simulink model "power_wind"  (R2014b)
settings: Solver=ode23tb  StartTime=0.0  StopTime=20  MaxStep=1/60  RelTol=1e-4  AbsTol=1e-3
InitFcn:
  | xInitial = init_power_wind_ig;
undefined symbols (not defined in the file): D1, D11, Delta
libraries: powerlib_meascontrol x45, powerlib x29, DRlib x3, factslib x1
(part 1 of 4)
Description:
  | Copyright 2008-2014 The MathWorks, Inc.
settings Model: ExtModeAutoUpdateStatusClock=off  Creator=MathWorks  LastModifiedBy=HPSEDC
settings DataIOCC: LoadInitialState=on  SignalLoggingSaveFormat=ModelDataLogs  SaveOutput=off  SaveTime=off  SignalLoggingName=logsOut
settings OptimizationCC: ExpressionDepthLimit=2147483647  InitFltsAndDblsToZero=on
settings DebuggingCC: UnderspecifiedInitializationDetection=Classic  MergeDetectMultiDrivingBlocksExec=none  CheckExecutionContextPreStartOutputMsg=on  CheckExecutionContextRuntimeOutputMsg=on  SignalResolutionControl=TryResolveAllWithWarning  MultiTaskDSMMsg=warning  MultiTaskCondExecSysMsg=none  FcnCallInpInsideContextMsg=UseLocalSettings  StateNameClashWarn=warning  InitInArrayFormatMsg=none
settings RTWCC: IncludeERTFirstTime=on
settings GRTTargetCC: CombineOutputUpdateFcns=off  GRTInterface=on

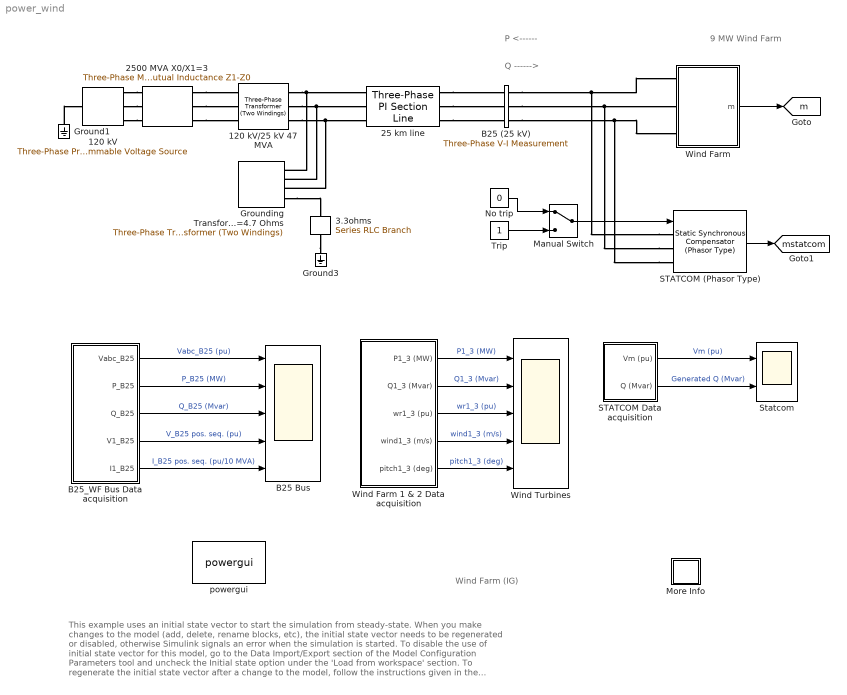
== system power_wind ==
  note: This example uses an initial state vector to start the simulation from steady-state. When you make changes to the model (add, delete, rename blocks, etc),
      | the initial state vector needs to be regenerated or disabled, otherwise Simulink signals an error when the simulation is started.
      | To disable the use of initial state vector for this model, go to the Data Import/Export section of the Model Configuration Parameters tool and uncheck the
      | Initial state option under the 'Load from workspace' section.
      | To regenerate the initial state vector after a change to the model, follow the instructions given in the initialization file for this model.
      | Type open('init_power_wind_ig') at the matlab prompt to view this file.
  note: Wind Farm (IG)
  note: P
      | <------
  note: Q
      | ------>
  note: 9 MW Wind Farm
  " Wind Turbines" : Scope  NumInputPorts=5
  120 kV : powerlib/Electrical Sources/Three-Phase Programmable Voltage Source  PositiveSequence=[120e3 0 60]  VariationEntity=None  VariationType=Table of time-amplitude pairs  VariationTypeAlt=Step  VariationStep=-0.15  VariationRate=10  VariationMagnitude=0.3  VariationFrequency=2  VariationTiming=[5 5.5]  VariationPhaseA=off  Amplitudes="[1.0  0.5  1.0 ]"  TimeValues="[0  10  10.1]"  HarmonicGeneration=off  HarmonicA=[1 -0.1 0 1]  HarmonicB=[2 0.15 35 2]  Timing="[5  5.5]"  BusType=swing  Pref=1e3  Qref=0  Qmin=-inf  Qmax=inf
  120 kV/25 kV 47 MVA : powerlib/Elements/Three-Phase Transformer (Two Windings)  Winding1Connection=Yg  UNITS=pu  NominalPower=[47e6 60 ]  Winding1="[ 120e3  0.08/30   0.08 ]"  Winding2Connection=Delta (D1)  Winding2="[ 25e3  0.08/30  0.08]"  SetSaturation=off  Rm=500  Lm=500  Saturation="[ 0,0  ;  0.005,1.2  ;  1.0,1.4 ]"  Hysteresis=off  DataFile='basic_model'  SetInitialFlux=off  InitialFluxes=[ 0.8 , -0.8 , 0.7 ]  Measurements=None  MoreParameters=off  BreakLoop=off  DataType=off  TransfoNumber=0
  25 km line : powerlib/Elements/Three-Phase PI Section Line  LConnTagsString=a|b|c  RConnTagsString=A|B|C  Frequency=60  Resistances=[0.1153 0.413]  Inductances=[1.05e-3 3.32e-3]  Capacitances=[11.33e-009 5.01e-009]  Length=25
  2500 MVA X0/X1=3 : powerlib/Elements/Three-Phase Mutual Inductance Z1-Z0  LConnTagsString=a|b|c  RConnTagsString=A|B|C  PositiveSequence="[0.1  1.0/(2*pi*60)] *120e3^2/2500e6"  ZeroSequence="[0.3  3.0/(2*pi*60)] *120e3^2/2500e6"
  "3.3ohms " : powerlib/Elements/Series RLC Branch  LConnTagsString=__new0  RConnTagsString=__new0  BranchType=R  Resistance=3.3  Inductance=1.0  SetiL0=off  InitialCurrent=0  Capacitance=1.0  Setx0=off  InitialVoltage=0  Measurements=None
  B25 (25 kV) : powerlib/Measurements/Three-Phase V-I Measurement  VoltageMeasurement=phase-to-ground  SetLabelV=on  LabelV=Vabc_B25  Vpu=on  VpuLL=off  CurrentMeasurement=yes  SetLabelI=on  LabelI=Iabc_B25  Ipu=on  Pbase=10e6  Vbase=25e3  OutputType=Complex  PhasorSimulation=on  PSBequivalent=0
  B25 Bus : Scope  NumInputPorts=5
  B25_WF Bus Data acquisition : Subsystem
  Ground1 : powerlib/Elements/Ground  LConnTagsString=a
  Ground3 : powerlib/Elements/Ground  LConnTagsString=a
  Grounding Transformer X0=4.7 Ohms : powerlib/Elements/Three-Phase Transformer (Two Windings)  Winding1Connection=Yn  UNITS=pu  NominalPower=[100e6 60]  Winding1="[ 25e3  4.7/(25e3^2/100e6)/30    4.7/(25e3^2/100e6)]"  Winding2Connection=Delta (D11)  Winding2="[ 25e3  1e-6  0]"  SetSaturation=off  Rm=500  Lm=500  Saturation="[ 0,0  ;  0.005,1.2  ;  1.0,1.4 ]"  Hysteresis=off  DataFile='basic_model'  SetInitialFlux=off  InitialFluxes=[ 0.8 , -0.8 , 0.7 ]  Measurements=None  MoreParameters=off  BreakLoop=off  DataType=off  TransfoNumber=0
  Manual Switch : ManualSwitch
  More Info : Subsystem
      settings: OpenFcn=showdemo(bdroot(gcb))
      mask Display: disp('?')
  No trip : Constant  Value=0
  STATCOM (Phasor Type) : factslib/Power-Electronics Based FACTS/Static Synchronous Compensator (Phasor Type)  ShowParameters=Power data  SystemNominal=[ 25e3, 60 ]  Pnom_SH=3e6  RL_SH=[ 0.22/30, 0.22 ]  Iinit_SH=[0, 0 ]  VnomDC=40000/10  C_DC=375e-6*(3/100)*10^2  OpMode_SH=Voltage regulation  ExternalVref=off  Vref_SH=1.00  MaxRateChangeVref_SH=10  Droop_SH=0.03  Par_VacReg=[5 1000]  Qref_SH=0  MaxRateChangeQref_SH=2  Par_VdcReg=[0.1e-3 20e-3]  Par_IReg_SH=[0.3 10 0.22]
  STATCOM Data acquisition : Subsystem
  Statcom : Scope  NumInputPorts=2
  Trip : Constant
  Wind Farm : Subsystem
      mask Display:
      | plot(0,0,118,100)
      | plot([56 62],[4 4],[56 57],[4 52],[62 61],[4 52])
      | plot([57 59 61],[52 52.5 52])
      | plot([61 61.5 62 63 63],[52 52.2 52.5 54 56])
      | plot([63 59 57.6 57.3 56 55],[56 58 57.8 55.6 54.2 54])
      | plot([55 57],[54 52],[57.3 63],[55.6 54])
      | plot([57.6 57 55 54.7 60 81],[57.6 57.3 58 59.4 64 82])
      | plot([81 83 84 84.2 83 81],[82 83.6 83.4 83 80.8 78.7])
      | plot([81 60.5 57.6],[78.7 60 57.6])
      | plot([54.7 53 51 51.3 52.5],[59.4 58.8 58 56 55])
      | plot([52.5 53.7 54.5 55],[55 54.9 54.6 54])
      | plot([51 47 35 33 32 33 35],[58 59 66 67.7 68.5 68.4 68])
      | plot([35 45 52 53 53.7],[68 64 61 60 59.2])
      | plot([52.5 51 50.8 51.5 55],[55 26 21 26 54])
  Wind Farm 1 & 2 Data acquisition : Subsystem
  powergui : powerlib/powergui  Priority=2  SimulationMode=Phasor  SolverType=Tustin  SampleTime=0  frequency=60  SPID=off  DisableSnubberDevices=off  DisableRonSwitches=off  DisableVfSwitches=off  SwTol=0  DisplayEquations=off  Interpol=off  methode=off  Ts=0  frequencyindice=60  Pbase=100e6  ErrMax=1e-4  Iterations=50  UnitsV=kV  UnitsW=MW  FunctionMessages=off  echomessages=off  HookPort=off  EnableUseOfTLC=off  x0status=blocks  RestoreLinks=no  ResistiveCurrentMeasurement=off  Frange=[0:2:500]  Ylog=off  Xlog=off  ShowGrid=off  save=off  variable=ZData  structure=0  ZoomFFT=on  StartTime=0.0  cycles=1  DisplayStyle=1  fundamental=60  FreqAxis=off  MaxFrequency=1000  frequencyindicesteady=1  RmsSteady=1  display=off
  tag scope: m=global, mstatcom=global
  wires:
  B25_WF Bus Data acquisition/1("Vabc_B25 ") -> B25 Bus/1  "Vabc_B25 (pu)"
  B25_WF Bus Data acquisition/2(P_B25) -> B25 Bus/2  "P_B25 (MW)"
  B25_WF Bus Data acquisition/3(Q_B25) -> B25 Bus/3  "Q_B25 (Mvar)"
  B25_WF Bus Data acquisition/4(V1_B25) -> B25 Bus/4  "V_B25 pos. seq. (pu)"
  B25_WF Bus Data acquisition/5(I1_B25) -> B25 Bus/5  "I_B25 pos. seq. (pu/10 MVA)"
  Wind Farm/1(m) -> [m]
  No trip/1 -> Manual Switch/1
  Trip/1 -> Manual Switch/2
  STATCOM Data acquisition/1(Vm (pu)) -> Statcom/1  "Vm (pu)"
  STATCOM Data acquisition/2(Q (Mvar)) -> Statcom/2  "Generated Q (Mvar)"
  Wind Farm 1 & 2 Data acquisition/1(P1_3 (MW)) -> " Wind Turbines"/1  "P1_3 (MW)"
  Wind Farm 1 & 2 Data acquisition/2(Q1_3 (Mvar)) -> " Wind Turbines"/2  "Q1_3 (Mvar)"
  Wind Farm 1 & 2 Data acquisition/3(wr1_3 (pu)) -> " Wind Turbines"/3  "wr1_3 (pu)"
  Wind Farm 1 & 2 Data acquisition/4(wind1_3 (m/s)) -> " Wind Turbines"/4  "wind1_3 (m/s)"
  Wind Farm 1 & 2 Data acquisition/5(pitch1_3 (deg)) -> " Wind Turbines"/5  "pitch1_3 (deg)"
  Manual Switch/1 -> STATCOM (Phasor Type)/1
  STATCOM (Phasor Type)/1 -> [mstatcom]
  connections:
  120 kV/25 kV 47 MVA/RConn2 -- 25 km line/LConn2 -- Grounding Transformer X0=4.7 Ohms/LConn2
  120 kV/25 kV 47 MVA/RConn3 -- 25 km line/LConn3 -- Grounding Transformer X0=4.7 Ohms/LConn3
  120 kV/25 kV 47 MVA/RConn1 -- 25 km line/LConn1 -- Grounding Transformer X0=4.7 Ohms/LConn1
  STATCOM (Phasor Type)/LConn2 -- B25 (25 kV)/RConn2 -- Wind Farm/LConn2
  STATCOM (Phasor Type)/LConn3 -- B25 (25 kV)/RConn3 -- Wind Farm/LConn3
  Ground1/LConn1 -- 120 kV/LConn1
  120 kV/RConn1 -- 2500 MVA X0/X1=3/LConn1
  120 kV/RConn2 -- 2500 MVA X0/X1=3/LConn2
  120 kV/RConn3 -- 2500 MVA X0/X1=3/LConn3
  "3.3ohms "/RConn1 -- Ground3/LConn1
  Grounding Transformer X0=4.7 Ohms/LConn4 -- "3.3ohms "/LConn1
  2500 MVA X0/X1=3/RConn1 -- 120 kV/25 kV 47 MVA/LConn1
  2500 MVA X0/X1=3/RConn2 -- 120 kV/25 kV 47 MVA/LConn2
  2500 MVA X0/X1=3/RConn3 -- 120 kV/25 kV 47 MVA/LConn3
  STATCOM (Phasor Type)/LConn1 -- B25 (25 kV)/RConn1 -- Wind Farm/LConn1
  25 km line/RConn1 -- B25 (25 kV)/LConn1
  25 km line/RConn2 -- B25 (25 kV)/LConn2
  25 km line/RConn3 -- B25 (25 kV)/LConn3

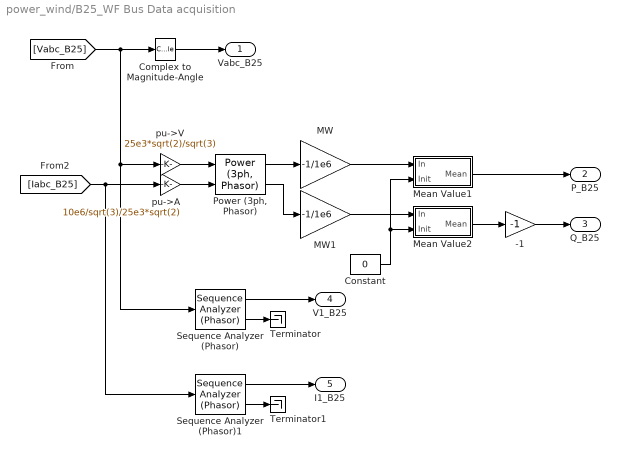
== system power_wind/B25_WF Bus Data acquisition ==
  -1 : Gain  Gain=-1  SaturateOnIntegerOverflow=on  OutDataTypeStr=Inherit: Same as input  ParamDataTypeStr=Inherit: Same as input
  "Complex to Magnitude-Angle " : ComplexToMagnitudeAngle  Output=Magnitude
  Constant : Constant  Value=0
  MW : Gain  Gain=-1/1e6  SaturateOnIntegerOverflow=on  OutDataTypeStr=Inherit: Same as input  ParamDataTypeStr=Inherit: Same as input
  MW1 : Gain  Gain=-1/1e6  SaturateOnIntegerOverflow=on  OutDataTypeStr=Inherit: Same as input  ParamDataTypeStr=Inherit: Same as input
  Mean Value1 : Subsystem  mask(Mean value){Period=1/60}
      mask prompts: Period "Averaging period (s):"
      mask help: This block uses the running window averaging technique to compute the mean value of the input signal over the specified period.
  Mean Value2 : Subsystem  mask(Mean value){Period=1/60}
      mask prompts: Period "Averaging period (s):"
      mask help: This block uses the running window averaging technique to compute the mean value of the input signal over the specified period.
  "Power (3ph, Phasor)" : powerlib_meascontrol/Measurements/Power (3ph, Phasor)
  Sequence Analyzer (Phasor) : powerlib_meascontrol/Measurements/Sequence Analyzer (Phasor)  seq=Positive
  Sequence Analyzer (Phasor)1 : powerlib_meascontrol/Measurements/Sequence Analyzer (Phasor)  seq=Positive
  Terminator : Terminator
  Terminator1 : Terminator
  pu->A : Gain  Gain=10e6/sqrt(3)/25e3*sqrt(2)  SaturateOnIntegerOverflow=on  OutDataTypeStr=Inherit: Same as input  ParamDataTypeStr=Inherit: Same as input
  pu->V : Gain  Gain=25e3*sqrt(2)/sqrt(3)  SaturateOnIntegerOverflow=on  OutDataTypeStr=Inherit: Same as input  ParamDataTypeStr=Inherit: Same as input
  "Vabc_B25 " : Outport
  P_B25 : Outport  Port=2
  Q_B25 : Outport  Port=3
  V1_B25 : Outport  Port=4
  I1_B25 : Outport  Port=5
  wires:
  pu->A/1 -> "Power (3ph, Phasor)"/2
  pu->V/1 -> "Power (3ph, Phasor)"/1
  "Power (3ph, Phasor)"/1 -> MW/1
  "Complex to Magnitude-Angle "/1 -> "Vabc_B25 "/1
  [Vabc_B25] -> Sequence Analyzer (Phasor)/1, pu->V/1, "Complex to Magnitude-Angle "/1
  [Iabc_B25] -> Sequence Analyzer (Phasor)1/1, pu->A/1
  MW/1 -> Mean Value1/1(In)
  MW1/1 -> Mean Value2/1(In)
  Constant/1 -> Mean Value1/2(Init), Mean Value2/2(Init)
  Mean Value1/1(Mean) -> P_B25/1
  Mean Value2/1(Mean) -> -1/1
  Sequence Analyzer (Phasor)/1 -> V1_B25/1
  Sequence Analyzer (Phasor)/2 -> Terminator/1
  Sequence Analyzer (Phasor)1/1 -> I1_B25/1
  Sequence Analyzer (Phasor)1/2 -> Terminator1/1
  -1/1 -> Q_B25/1
  "Power (3ph, Phasor)"/2 -> MW1/1

== system power_wind/More Info ==

== system power_wind/STATCOM Data acquisition ==
  Bus Selector : BusSelector  OutputSignals=Control.Vm (pu),Control.Qm (pu)
  pu->Mvar : Gain  Gain=-3e6/1e6  SaturateOnIntegerOverflow=on  OutDataTypeStr=Inherit: Same as input  ParamDataTypeStr=Inherit: Same as input
  Vm (pu) : Outport
  Q (Mvar) : Outport  Port=2
  wires:
  Bus Selector/1 -> Vm (pu)/1  "<Vm (pu)>"
  Bus Selector/2 -> pu->Mvar/1  "<Qm (pu)>"
  pu->Mvar/1 -> Q (Mvar)/1  "Generated Q (Mvar)"
  [mstatcom] -> Bus Selector/1

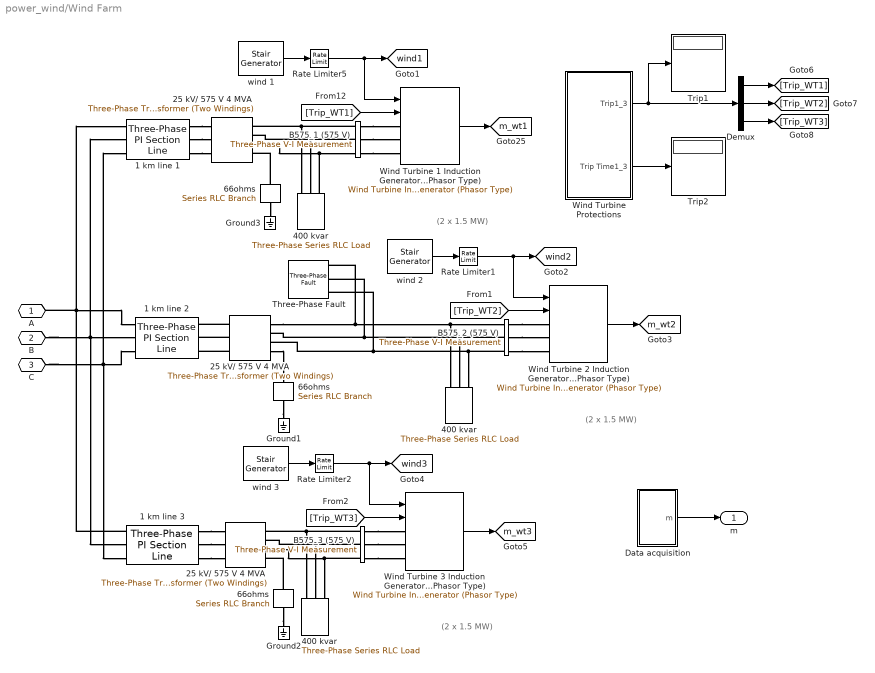
== system power_wind/Wind Farm ==
  note: (2 x 1.5 MW)
  note: (2 x 1.5 MW)
  note: (2 x 1.5 MW)
  " 66ohms " : powerlib/Elements/Series RLC Branch  LConnTagsString=__new0  RConnTagsString=__new0  BranchType=R  Resistance=66  Inductance=1.0  SetiL0=off  InitialCurrent=0  Capacitance=1.0  Setx0=off  InitialVoltage=0  Measurements=None
  "1 km line 1 " : powerlib/Elements/Three-Phase PI Section Line  LConnTagsString=a|b|c  RConnTagsString=A|B|C  Frequency=60  Resistances=[0.1153 0.413]  Inductances=[1.05e-3 3.32e-3]  Capacitances=[11.33e-009 5.01e-009]  Length=1
  1 km line 2 : powerlib/Elements/Three-Phase PI Section Line  LConnTagsString=a|b|c  RConnTagsString=A|B|C  Frequency=60  Resistances=[0.1153 0.413]  Inductances=[1.05e-3 3.32e-3]  Capacitances=[11.33e-009 5.01e-009]  Length=1
  1 km line 3 : powerlib/Elements/Three-Phase PI Section Line  LConnTagsString=a|b|c  RConnTagsString=A|B|C  Frequency=60  Resistances=[0.1153 0.413]  Inductances=[1.05e-3 3.32e-3]  Capacitances=[11.33e-009 5.01e-009]  Length=1
  25 kV/ 575 V 4 MVA : powerlib/Elements/Three-Phase Transformer (Two Windings)  Winding1Connection=Yg  UNITS=pu  NominalPower="[4e6  60]"  Winding1=[25e3 , 0.025/30 , 0.025]  Winding2Connection=Yn  Winding2=[ 575, 0.025/30 , 0.025]  SetSaturation=off  Rm=500  Lm=inf  Saturation=[ 0,0 ; 0.0024,1.2 ; 1.0,1.52 ]  Hysteresis=off  DataFile='hysteresis'  SetInitialFlux=off  InitialFluxes=[ 0.8 , -0.8 , 0.7 ]  Measurements=None  MoreParameters=off  BreakLoop=off  DataType=off  TransfoNumber=0
  "25 kV/ 575 V 4 MVA " : powerlib/Elements/Three-Phase Transformer (Two Windings)  Winding1Connection=Yg  UNITS=pu  NominalPower="[4e6  60]"  Winding1=[25e3 , 0.025/30 , 0.025]  Winding2Connection=Yn  Winding2=[ 575, 0.025/30 , 0.025]  SetSaturation=off  Rm=500  Lm=inf  Saturation=[ 0,0 ; 0.0024,1.2 ; 1.0,1.52 ]  Hysteresis=off  DataFile='hysteresis'  SetInitialFlux=off  InitialFluxes=[ 0.8 , -0.8 , 0.7 ]  Measurements=None  MoreParameters=off  BreakLoop=off  DataType=off  TransfoNumber=0
  "25 kV/ 575 V 4 MVA  " : powerlib/Elements/Three-Phase Transformer (Two Windings)  Winding1Connection=Yg  UNITS=pu  NominalPower="[4e6  60]"  Winding1=[25e3 , 0.025/30 , 0.025]  Winding2Connection=Yn  Winding2=[ 575, 0.025/30 , 0.025]  SetSaturation=off  Rm=500  Lm=inf  Saturation=[ 0,0 ; 0.0024,1.2 ; 1.0,1.52 ]  Hysteresis=off  DataFile='hysteresis'  SetInitialFlux=off  InitialFluxes=[ 0.8 , -0.8 , 0.7 ]  Measurements=None  MoreParameters=off  BreakLoop=off  DataType=off  TransfoNumber=0
  400 kvar : powerlib/Elements/Three-Phase Series RLC Load  LConnTagsString=A|B|C  Configuration=Delta  NominalVoltage=575  NominalFrequency=60  ActivePower=0  InductivePower=0  CapacitivePower=400e3  Measurements=None  LoadType=constant Z
  "400 kvar " : powerlib/Elements/Three-Phase Series RLC Load  LConnTagsString=A|B|C  Configuration=Delta  NominalVoltage=575  NominalFrequency=60  ActivePower=0  InductivePower=0  CapacitivePower=400e3  Measurements=None  LoadType=constant Z
  "400 kvar  " : powerlib/Elements/Three-Phase Series RLC Load  LConnTagsString=A|B|C  Configuration=Delta  NominalVoltage=575  NominalFrequency=60  ActivePower=0  InductivePower=0  CapacitivePower=400e3  Measurements=None  LoadType=constant Z
  "66ohms " : powerlib/Elements/Series RLC Branch  LConnTagsString=__new0  RConnTagsString=__new0  BranchType=R  Resistance=66  Inductance=1.0  SetiL0=off  InitialCurrent=0  Capacitance=1.0  Setx0=off  InitialVoltage=0  Measurements=None
  "66ohms  " : powerlib/Elements/Series RLC Branch  LConnTagsString=__new0  RConnTagsString=__new0  BranchType=R  Resistance=66  Inductance=1.0  SetiL0=off  InitialCurrent=0  Capacitance=1.0  Setx0=off  InitialVoltage=0  Measurements=None
  B575_1 (575 V) : powerlib/Measurements/Three-Phase V-I Measurement  VoltageMeasurement=phase-to-ground  SetLabelV=on  LabelV=Vabc_B575_1  Vpu=on  VpuLL=off  CurrentMeasurement=yes  SetLabelI=on  LabelI=Iabc_B575_1  Ipu=on  Pbase=2*1.5e6/0.9  Vbase=575  OutputType=Complex  PhasorSimulation=on  PSBequivalent=0
  B575_2 (575 V) : powerlib/Measurements/Three-Phase V-I Measurement  VoltageMeasurement=phase-to-ground  SetLabelV=on  LabelV=Vabc_B575_2  Vpu=on  VpuLL=off  CurrentMeasurement=yes  SetLabelI=on  LabelI=Iabc_B575_2  Ipu=on  Pbase=2*1.5e6/0.9  Vbase=575  OutputType=Complex  PhasorSimulation=on  PSBequivalent=0
  B575_3 (575 V) : powerlib/Measurements/Three-Phase V-I Measurement  VoltageMeasurement=phase-to-ground  SetLabelV=on  LabelV=Vabc_B575_3  Vpu=on  VpuLL=off  CurrentMeasurement=yes  SetLabelI=on  LabelI=Iabc_B575_3  Ipu=on  Pbase=2*1.5e6/0.9  Vbase=575  OutputType=Complex  PhasorSimulation=on  PSBequivalent=0
  Data acquisition : Subsystem
  Demux : Demux  Outputs=3
  Ground1 : powerlib/Elements/Ground  LConnTagsString=a
  Ground2 : powerlib/Elements/Ground  LConnTagsString=a
  Ground3 : powerlib/Elements/Ground  LConnTagsString=a
  Rate Limiter1 : RateLimiter
  Rate Limiter2 : RateLimiter
  Rate Limiter5 : RateLimiter
  Three-Phase Fault : powerlib/Elements/Three-Phase Fault  InitialStates=0  FaultA=on  FaultB=on  FaultC=off  GroundFault=on  SwitchTimes=[ 15 15.1]  External=off  SwitchStatus=NaN  FaultResistance=0.001  GroundResistance=0.001  SnubberResistance=1e6  SnubberCapacitance=inf  Measurements=None
  Trip1 : Display
  Trip2 : Display
  Wind Turbine Protections : Subsystem
  Wind Turbine 1 Induction Generator (Phasor Type) : DRlib/Wind Generation/Wind Turbine Induction Generator (Phasor Type)  ShowParameters=Turbine data  nom=[2*1.5e6/0.9 575 60]  sta=[ 0.004843 0.1248]  rot=[ 0.004377 0.1791]  Lm=6.77  mec=[5.04 0.01 3]  init="[ -0.01,0   0,0,0   0,0,0 ]"  ExternalTm=off  DisplayTurbChar=off  pitch_angle=0  Pmec=2*1.5e6  wind_base=9  P_wind_base=1  speed_nom=1  K_pitch_gain=[5 25]  pitch_max=45  pitch_rate=2
  Wind Turbine 2 Induction Generator (Phasor Type) : DRlib/Wind Generation/Wind Turbine Induction Generator (Phasor Type)  ShowParameters=Turbine data  nom=[2*1.5e6/0.9 575 60]  sta=[ 0.004843 0.1248]  rot=[ 0.004377 0.1791]  Lm=6.77  mec=[5.04 0.01 3]  init="[ -0.01,0   0,0,0   0,0,0 ]"  ExternalTm=off  DisplayTurbChar=off  pitch_angle=0  Pmec=2*1.5e6  wind_base=9  P_wind_base=1  speed_nom=1  K_pitch_gain=[5 25]  pitch_max=45  pitch_rate=2
  Wind Turbine 3 Induction Generator (Phasor Type) : DRlib/Wind Generation/Wind Turbine Induction Generator (Phasor Type)  ShowParameters=Turbine data  nom=[2*1.5e6/0.9 575 60]  sta=[ 0.004843 0.1248]  rot=[ 0.004377 0.1791]  Lm=6.77  mec=[5.04 0.01 3]  init="[ -0.01,0   0,0,0   0,0,0 ]"  ExternalTm=off  DisplayTurbChar=off  pitch_angle=0  Pmec=2*1.5e6  wind_base=9  P_wind_base=1  speed_nom=1  K_pitch_gain=[5 25]  pitch_max=45  pitch_rate=2
  wind 1 : powerlib_meascontrol/Pulse & Signal Generators/Stair Generator  t=[ 0 2]  e=[8 11]  Ts=0
  wind 2 : powerlib_meascontrol/Pulse & Signal Generators/Stair Generator  t=[ 0 4]  e=[8 11]  Ts=0
  wind 3 : powerlib_meascontrol/Pulse & Signal Generators/Stair Generator  t=[ 0 6]  e=[8 11]  Ts=0
  A : PMIOPort  Port=1  Side=Left
  B : PMIOPort  Port=2  Side=Left
  C : PMIOPort  Port=3  Side=Left
  m : Outport
  tag scope: m_wt1=global, m_wt2=global, m_wt3=global, wind1=global, wind2=global, wind3=global
  wires:
  Data acquisition/1(m) -> m/1
  Wind Turbine 1 Induction Generator (Phasor Type)/1 -> [m_wt1]
  Rate Limiter5/1 -> [wind1], Wind Turbine 1 Induction Generator (Phasor Type)/1
  wind 1/1 -> Rate Limiter5/1
  [Trip_WT1] -> Wind Turbine 1 Induction Generator (Phasor Type)/2
  Wind Turbine 2 Induction Generator (Phasor Type)/1 -> [m_wt2]
  Rate Limiter1/1 -> Wind Turbine 2 Induction Generator (Phasor Type)/1, [wind2]
  wind 2/1 -> Rate Limiter1/1
  [Trip_WT2] -> Wind Turbine 2 Induction Generator (Phasor Type)/2
  Wind Turbine 3 Induction Generator (Phasor Type)/1 -> [m_wt3]
  Rate Limiter2/1 -> [wind3], Wind Turbine 3 Induction Generator (Phasor Type)/1
  wind 3/1 -> Rate Limiter2/1
  [Trip_WT3] -> Wind Turbine 3 Induction Generator (Phasor Type)/2
  Wind Turbine Protections/1(Trip1_3) -> Trip1/1, Demux/1
  Demux/1 -> [Trip_WT1]
  Wind Turbine Protections/2(Trip Time1_3) -> Trip2/1
  Demux/2 -> [Trip_WT2]
  Demux/3 -> [Trip_WT3]
  connections:
  B575_1 (575 V)/RConn3 -- Wind Turbine 1 Induction Generator (Phasor Type)/LConn3
  B575_1 (575 V)/RConn2 -- Wind Turbine 1 Induction Generator (Phasor Type)/LConn2
  B575_1 (575 V)/RConn1 -- Wind Turbine 1 Induction Generator (Phasor Type)/LConn1
  400 kvar/LConn3 -- B575_1 (575 V)/LConn3 -- 25 kV/ 575 V 4 MVA/RConn3
  25 kV/ 575 V 4 MVA/RConn2 -- 400 kvar/LConn2 -- B575_1 (575 V)/LConn2
  25 kV/ 575 V 4 MVA/RConn1 -- 400 kvar/LConn1 -- B575_1 (575 V)/LConn1
  "1 km line 1 "/RConn3 -- 25 kV/ 575 V 4 MVA/LConn3
  "1 km line 1 "/RConn2 -- 25 kV/ 575 V 4 MVA/LConn2
  "1 km line 1 "/RConn1 -- 25 kV/ 575 V 4 MVA/LConn1
  Three-Phase Fault/LConn3 -- "400 kvar "/LConn3 -- B575_2 (575 V)/LConn3 -- "25 kV/ 575 V 4 MVA "/RConn3
  Three-Phase Fault/LConn2 -- "400 kvar "/LConn2 -- B575_2 (575 V)/LConn2 -- "25 kV/ 575 V 4 MVA "/RConn2
  Three-Phase Fault/LConn1 -- "25 kV/ 575 V 4 MVA "/RConn1 -- "400 kvar "/LConn1 -- B575_2 (575 V)/LConn1
  B575_2 (575 V)/RConn3 -- Wind Turbine 2 Induction Generator (Phasor Type)/LConn3
  B575_2 (575 V)/RConn2 -- Wind Turbine 2 Induction Generator (Phasor Type)/LConn2
  B575_2 (575 V)/RConn1 -- Wind Turbine 2 Induction Generator (Phasor Type)/LConn1
  "25 kV/ 575 V 4 MVA "/LConn3 -- 1 km line 2/RConn3
  "25 kV/ 575 V 4 MVA "/LConn2 -- 1 km line 2/RConn2
  "25 kV/ 575 V 4 MVA "/LConn1 -- 1 km line 2/RConn1
  B575_3 (575 V)/LConn3 -- "400 kvar  "/LConn3 -- "25 kV/ 575 V 4 MVA  "/RConn3
  "25 kV/ 575 V 4 MVA  "/RConn2 -- "400 kvar  "/LConn2 -- B575_3 (575 V)/LConn2
  "25 kV/ 575 V 4 MVA  "/RConn1 -- "400 kvar  "/LConn1 -- B575_3 (575 V)/LConn1
  B575_3 (575 V)/RConn3 -- Wind Turbine 3 Induction Generator (Phasor Type)/LConn3
  B575_3 (575 V)/RConn2 -- Wind Turbine 3 Induction Generator (Phasor Type)/LConn2
  B575_3 (575 V)/RConn1 -- Wind Turbine 3 Induction Generator (Phasor Type)/LConn1
  1 km line 3/RConn3 -- "25 kV/ 575 V 4 MVA  "/LConn3
  1 km line 3/RConn2 -- "25 kV/ 575 V 4 MVA  "/LConn2
  1 km line 3/RConn1 -- "25 kV/ 575 V 4 MVA  "/LConn1
  1 km line 3/LConn1 -- A/RConn1 -- "1 km line 1 "/LConn1 -- 1 km line 2/LConn1
  B/RConn1 -- "1 km line 1 "/LConn2 -- 1 km line 3/LConn2 -- 1 km line 2/LConn2
  C/RConn1 -- "1 km line 1 "/LConn3 -- 1 km line 3/LConn3 -- 1 km line 2/LConn3
  "66ohms "/RConn1 -- Ground3/LConn1
  "66ohms  "/RConn1 -- Ground1/LConn1
  "25 kV/ 575 V 4 MVA "/RConn4 -- "66ohms  "/LConn1
  " 66ohms "/RConn1 -- Ground2/LConn1
  " 66ohms "/LConn1 -- "25 kV/ 575 V 4 MVA  "/RConn4
  "66ohms "/LConn1 -- 25 kV/ 575 V 4 MVA/RConn4

== system power_wind/Wind Farm 1 & 2 Data acquisition ==
  -1 : Gain  Gain=-1  SaturateOnIntegerOverflow=on  OutDataTypeStr=Inherit: Same as input  ParamDataTypeStr=Inherit: Same as input
  Bus Selector1 : BusSelector  OutputSignals=P1_3 (MW),Q1_3 (Mvar),wr1_3,wind1_3 (m_s),pitch1_3
  Constant1 : Constant  Value=0
  Mean Value3 : Subsystem  mask(Mean value){Period=1/60}
      mask prompts: Period "Averaging period (s):"
      mask help: This block uses the running window averaging technique to compute the mean value of the input signal over the specified period.
  Mean Value4 : Subsystem  mask(Mean value){Period=1/60}
      mask prompts: Period "Averaging period (s):"
      mask help: This block uses the running window averaging technique to compute the mean value of the input signal over the specified period.
  P1_3 (MW) : Outport
  Q1_3 (Mvar) : Outport  Port=2
  wr1_3 (pu) : Outport  Port=3
  wind1_3 (m/s) : Outport  Port=4
  pitch1_3 (deg) : Outport  Port=5
  wires:
  [m] -> Bus Selector1/1
  Constant1/1 -> Mean Value4/2(Init), Mean Value3/2(Init)
  Mean Value4/1(Mean) -> -1/1
  Mean Value3/1(Mean) -> P1_3 (MW)/1
  -1/1 -> Q1_3 (Mvar)/1
  Bus Selector1/1 -> Mean Value3/1(In)  "<P1_3 (MW)>"
  Bus Selector1/2 -> Mean Value4/1(In)  "<Q1_3 (Mvar)>"
  Bus Selector1/3 -> wr1_3 (pu)/1  "<wr1_3>"
  Bus Selector1/4 -> wind1_3 (m/s)/1  "<wind1_3 (m_s)>"
  Bus Selector1/5 -> pitch1_3 (deg)/1  "<pitch1_3>"

== system power_wind/B25_WF Bus Data acquisition/Mean Value1 ==
  note: Mean value
  In : Inport
  Init : Inport  Port=2
  Gain : Gain  Gain=1/Period  SaturateOnIntegerOverflow=on  OutDataTypeStr=Inherit: Same as input  ParamDataTypeStr=Inherit: Same as input
  Step : Step  Time=Period+eps  SampleTime=0
  Sum : Sum  Inputs=+-  SaturateOnIntegerOverflow=on  InputSameDT=on  OutDataTypeStr=Inherit: Same as first input
  Switch : Switch  Threshold=0.5  SaturateOnIntegerOverflow=on
  Transport Delay : TransportDelay  DelayTime=Period
  integrator : Integrator
  Mean : Outport
  wires:
  Transport Delay/1 -> Sum/2
  integrator/1 -> Transport Delay/1, Sum/1
  In/1 -> integrator/1
  Sum/1 -> Gain/1
  Gain/1 -> Switch/1
  Switch/1 -> Mean/1
  Step/1 -> Switch/2
  Init/1 -> Switch/3

== system power_wind/B25_WF Bus Data acquisition/Mean Value2 ==
  note: Mean value
  In : Inport
  Init : Inport  Port=2
  Gain : Gain  Gain=1/Period  SaturateOnIntegerOverflow=on  OutDataTypeStr=Inherit: Same as input  ParamDataTypeStr=Inherit: Same as input
  Step : Step  Time=Period+eps  SampleTime=0
  Sum : Sum  Inputs=+-  SaturateOnIntegerOverflow=on  InputSameDT=on  OutDataTypeStr=Inherit: Same as first input
  Switch : Switch  Threshold=0.5  SaturateOnIntegerOverflow=on
  Transport Delay : TransportDelay  DelayTime=Period
  integrator : Integrator
  Mean : Outport
  wires:
  Init/1 -> Switch/3
  Step/1 -> Switch/2
  Switch/1 -> Mean/1
  Gain/1 -> Switch/1
  Sum/1 -> Gain/1
  In/1 -> integrator/1
  integrator/1 -> Sum/1, Transport Delay/1
  Transport Delay/1 -> Sum/2

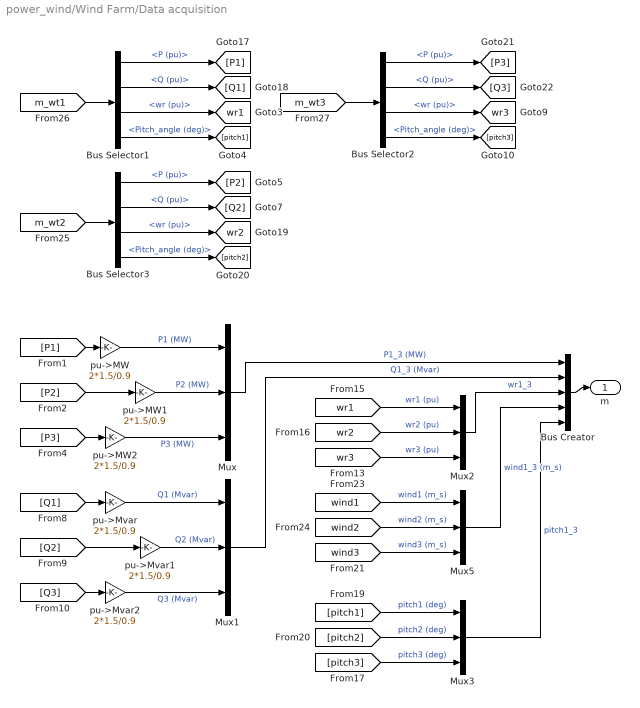
== system power_wind/Wind Farm/Data acquisition ==
  Bus Creator : BusCreator  Inputs=5
  Bus Selector1 : BusSelector  OutputSignals=P (pu),Q (pu),wr (pu),Pitch_angle (deg)
  Bus Selector2 : BusSelector  OutputSignals=P (pu),Q (pu),wr (pu),Pitch_angle (deg)
  Bus Selector3 : BusSelector  OutputSignals=P (pu),Q (pu),wr (pu),Pitch_angle (deg)
  Mux{,1..3,5} (5 alike) : Mux  Inputs=3
  pu->MW : Gain  Gain=2*1.5/0.9  SaturateOnIntegerOverflow=on  OutDataTypeStr=Inherit: Same as input  ParamDataTypeStr=Inherit: Same as input
  pu->MW1 : Gain  Gain=2*1.5/0.9  SaturateOnIntegerOverflow=on  OutDataTypeStr=Inherit: Same as input  ParamDataTypeStr=Inherit: Same as input
  pu->MW2 : Gain  Gain=2*1.5/0.9  SaturateOnIntegerOverflow=on  OutDataTypeStr=Inherit: Same as input  ParamDataTypeStr=Inherit: Same as input
  pu->Mvar : Gain  Gain=2*1.5/0.9  SaturateOnIntegerOverflow=on  OutDataTypeStr=Inherit: Same as input  ParamDataTypeStr=Inherit: Same as input
  pu->Mvar1 : Gain  Gain=2*1.5/0.9  SaturateOnIntegerOverflow=on  OutDataTypeStr=Inherit: Same as input  ParamDataTypeStr=Inherit: Same as input
  pu->Mvar2 : Gain  Gain=2*1.5/0.9  SaturateOnIntegerOverflow=on  OutDataTypeStr=Inherit: Same as input  ParamDataTypeStr=Inherit: Same as input
  m : Outport
  tag scope: wr1=global, wr2=global, wr3=global
  wires:
  [m_wt3] -> Bus Selector2/1
  [m_wt1] -> Bus Selector1/1
  [m_wt2] -> Bus Selector3/1
  Bus Selector1/2 -> [Q1]  "<Q (pu)>"
  Bus Selector1/1 -> [P1]  "<P (pu)>"
  Bus Selector1/4 -> [pitch1]  "<Pitch_angle (deg)>"
  Bus Selector1/3 -> [wr1]  "<wr (pu)>"
  Bus Selector3/4 -> [pitch2]  "<Pitch_angle (deg)>"
  Bus Selector3/3 -> [wr2]  "<wr (pu)>"
  Bus Selector3/2 -> [Q2]  "<Q (pu)>"
  Bus Selector2/4 -> [pitch3]  "<Pitch_angle (deg)>"
  Bus Selector2/3 -> [wr3]  "<wr (pu)>"
  Bus Selector2/2 -> [Q3]  "<Q (pu)>"
  Bus Selector2/1 -> [P3]  "<P (pu)>"
  Bus Selector3/1 -> [P2]  "<P (pu)>"
  Mux5/1 -> Bus Creator/4  "wind1_3 (m_s)"
  Mux3/1 -> Bus Creator/5  "pitch1_3"
  [wind3] -> Mux5/3  "wind3 (m_s)"
  [wind2] -> Mux5/2  "wind2 (m_s)"
  [wind1] -> Mux5/1  "wind1 (m_s)"
  Bus Creator/1 -> m/1
  Mux2/1 -> Bus Creator/3  "wr1_3"
  Mux1/1 -> Bus Creator/2  "Q1_3 (Mvar)"
  Mux/1 -> Bus Creator/1  "P1_3 (MW)"
  pu->Mvar2/1 -> Mux1/3  "Q3 (Mvar)"
  pu->Mvar1/1 -> Mux1/2  "Q2 (Mvar)"
  pu->Mvar/1 -> Mux1/1  "Q1 (Mvar)"
  [Q1] -> pu->Mvar/1
  [Q2] -> pu->Mvar1/1
  [Q3] -> pu->Mvar2/1
  pu->MW2/1 -> Mux/3  "P3 (MW)"
  pu->MW1/1 -> Mux/2  "P2 (MW)"
  pu->MW/1 -> Mux/1  "P1 (MW)"
  [pitch3] -> Mux3/3  "pitch3 (deg)"
  [pitch2] -> Mux3/2  "pitch2 (deg)"
  [pitch1] -> Mux3/1  "pitch1 (deg)"
  [wr3] -> Mux2/3  "wr3 (pu)"
  [wr2] -> Mux2/2  "wr2 (pu)"
  [wr1] -> Mux2/1  "wr1 (pu)"
  [P3] -> pu->MW2/1
  [P2] -> pu->MW1/1
  [P1] -> pu->MW/1

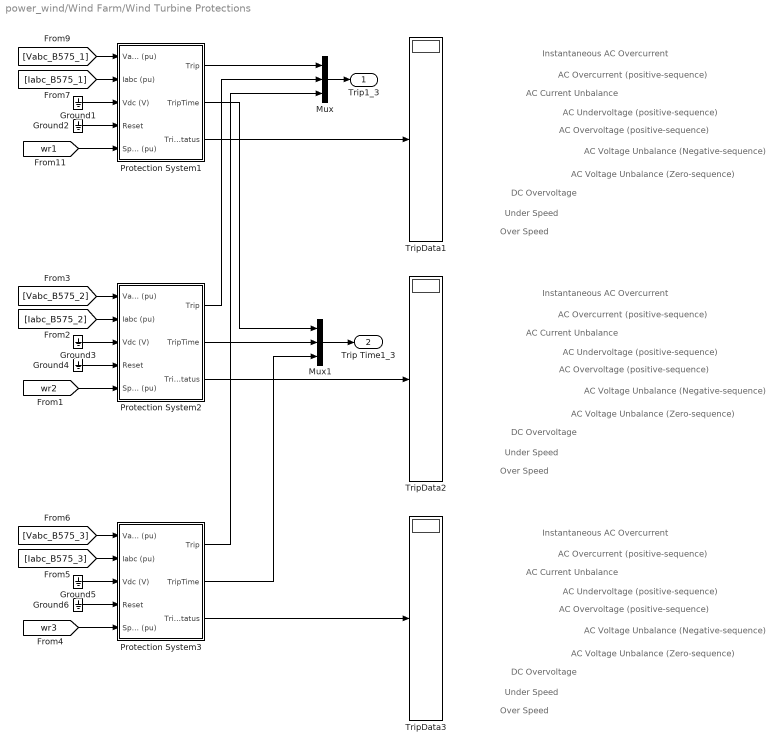
== system power_wind/Wind Farm/Wind Turbine Protections ==
  note: Under Speed
  note: DC Overvoltage
  note: AC Voltage Unbalance (Zero-sequence)
  note: AC Overvoltage (positive-sequence)
  note: AC Undervoltage (positive-sequence)
  note: AC Current Unbalance
  note: AC Overcurrent (positive-sequence)
  note: Instantaneous AC Overcurrent
  note: AC Voltage Unbalance (Negative-sequence)
  note: Over Speed
  note: Under Speed
  note: DC Overvoltage
  note: AC Voltage Unbalance (Zero-sequence)
  note: AC Overvoltage (positive-sequence)
  note: AC Undervoltage (positive-sequence)
  note: AC Current Unbalance
  note: AC Overcurrent (positive-sequence)
  note: Instantaneous AC Overcurrent
  note: AC Voltage Unbalance (Negative-sequence)
  note: Over Speed
  note: Under Speed
  note: DC Overvoltage
  note: AC Voltage Unbalance (Zero-sequence)
  note: AC Overvoltage (positive-sequence)
  note: AC Undervoltage (positive-sequence)
  note: AC Current Unbalance
  note: AC Overcurrent (positive-sequence)
  note: Instantaneous AC Overcurrent
  note: AC Voltage Unbalance (Negative-sequence)
  note: Over Speed
  Ground{1..6} (6 alike) : Ground
  Mux : Mux  Inputs=3
  Mux1 : Mux  Inputs=3
  Protection System1 : Subsystem  mask(Protection System){Freq=60, Max_Iinst=10, MaxI1=[ 1.1, 10 ], MaxI2I1=[ 0.4, 0.2], MinMaxV1=[ 0.75, 1.1, 0.1 ], MaxV2V1=[ 0.05, 0.05, 0.2 ], MaxVdc=[ 1900, 0.001 ], MaxSpeed=[ 1, 1.05, 5 ], Delay_Protection=5}
      mask prompts: Freq "Fundamental frequency f1 (Hz):"; Max_Iinst "Instantaneous AC Overcurrent (pu):"; MaxI1 "Maximum AC Current [ I1max(pu), Delay(s) ]:"; MaxI2I1 "Maximum AC Current Unbalance [ I2/I1max(pu), Delay(s) ]"; MinMaxV1 "AC Under/Over Voltage [ V1min(pu), V1max(pu), Delay(s) ]:"; MaxV2V1 "Maximum Voltage Unbalance [ V2/V1max(pu), V0/V1max(pu), Delay(s)]:"; MaxVdc "Maximum DC Voltage  [ Vmax(V), Delay(s) ]:"; MaxSpeed "Under/Over Speed [ Speedmin (pu), Speedmax (pu), Delay(s)]:"; Delay_Protection "Start time for protection system (s):"
      mask help:
      | Protection type:
      | 1.    Instantaneous AC Overcurrent
      | 2.    AC Overcurrent (positive-sequence)
      | 3.    AC Current Unbalance
      | 4.    AC Undervoltage (positive-sequence)
      | 5.    AC Overvoltage (positive-sequence)
      | 6.    AC Voltage Unbalance (Negative-sequence)
      | 7.    AC Voltage Unbalance (Zero-sequence)
      | 8.    DC Overvoltage
      | 9.    Under Speed
      | 10.  Over Speed
      mask init:
      | a=exp(2*pi*j/3);
      | a2=a^2;
      | Max_I1=MaxI1(1);
      | Delay_I1=MaxI1(2);
      | Max_I2_I1=MaxI2I1(1);
      | Delay_I2_I1=MaxI2I1(2);
      | Min_V1=MinMaxV1(1);
      | Max_V1=MinMaxV1(2);
      | Delay_V1=MinMaxV1(3);
      | Max_V2_V1=MaxV2V1(1);
      | Max_V0_V1=MaxV2V1(2);
      | Delay_V2_V1=MaxV2V1(3);
      | Max_Vdc=MaxVdc(1);
      | Delay_Vdc=MaxVdc(2);
      | Min_Speed=MaxSpeed(1);
      | Max_Speed=MaxSpeed(2);
      | Delay_Speed=MaxSpeed(3);
  Protection System2 : Subsystem  mask(Protection System){Freq=60, Max_Iinst=10, MaxI1=[ 1.1, 10 ], MaxI2I1=[ 0.4, 0.2], MinMaxV1=[ 0.75, 1.1, 0.1 ], MaxV2V1=[ 0.05, 0.05, 0.2 ], MaxVdc=[ 1900, 0.001 ], MaxSpeed=[ 1, 1.05, 5 ], Delay_Protection=5}
      mask prompts: Freq "Fundamental frequency f1 (Hz):"; Max_Iinst "Instantaneous AC Overcurrent (pu):"; MaxI1 "Maximum AC Current [ I1max(pu), Delay(s) ]:"; MaxI2I1 "Maximum AC Current Unbalance [ I2/I1max(pu), Delay(s) ]"; MinMaxV1 "AC Under/Over Voltage [ V1min(pu), V1max(pu), Delay(s) ]:"; MaxV2V1 "Maximum Voltage Unbalance [ V2/V1max(pu), V0/V1max(pu), Delay(s)]:"; MaxVdc "Maximum DC Voltage  [ Vmax(V), Delay(s) ]:"; MaxSpeed "Under/Over Speed [ Speedmin (pu), Speedmax (pu), Delay(s)]:"; Delay_Protection "Start time for protection system (s):"
      mask help:
      | Protection type:
      | 1.    Instantaneous AC Overcurrent
      | 2.    AC Overcurrent (positive-sequence)
      | 3.    AC Current Unbalance
      | 4.    AC Undervoltage (positive-sequence)
      | 5.    AC Overvoltage (positive-sequence)
      | 6.    AC Voltage Unbalance (Negative-sequence)
      | 7.    AC Voltage Unbalance (Zero-sequence)
      | 8.    DC Overvoltage
      | 9.    Under Speed
      | 10.  Over Speed
      mask init: same as power_wind/Wind Farm/Wind Turbine Protections/Protection System1
  Protection System3 : Subsystem  mask(Protection System){Freq=60, Max_Iinst=10, MaxI1=[ 1.1, 10 ], MaxI2I1=[ 0.4, 0.2], MinMaxV1=[ 0.75, 1.1, 0.1 ], MaxV2V1=[ 0.05, 0.05, 0.2 ], MaxVdc=[ 1900, 0.001 ], MaxSpeed=[ 1, 1.05, 5 ], Delay_Protection=5}
      mask prompts: Freq "Fundamental frequency f1 (Hz):"; Max_Iinst "Instantaneous AC Overcurrent (pu):"; MaxI1 "Maximum AC Current [ I1max(pu), Delay(s) ]:"; MaxI2I1 "Maximum AC Current Unbalance [ I2/I1max(pu), Delay(s) ]"; MinMaxV1 "AC Under/Over Voltage [ V1min(pu), V1max(pu), Delay(s) ]:"; MaxV2V1 "Maximum Voltage Unbalance [ V2/V1max(pu), V0/V1max(pu), Delay(s)]:"; MaxVdc "Maximum DC Voltage  [ Vmax(V), Delay(s) ]:"; MaxSpeed "Under/Over Speed [ Speedmin (pu), Speedmax (pu), Delay(s)]:"; Delay_Protection "Start time for protection system (s):"
      mask help:
      | Protection type:
      | 1.    Instantaneous AC Overcurrent
      | 2.    AC Overcurrent (positive-sequence)
      | 3.    AC Current Unbalance
      | 4.    AC Undervoltage (positive-sequence)
      | 5.    AC Overvoltage (positive-sequence)
      | 6.    AC Voltage Unbalance (Negative-sequence)
      | 7.    AC Voltage Unbalance (Zero-sequence)
      | 8.    DC Overvoltage
      | 9.    Under Speed
      | 10.  Over Speed
      mask init: same as power_wind/Wind Farm/Wind Turbine Protections/Protection System1
  TripData1 : Display
  TripData2 : Display
  TripData3 : Display
  Trip1_3 : Outport
  Trip Time1_3 : Outport  Port=2
  wires:
  Ground1/1 -> Protection System1/3(Vdc (V))
  Protection System1/2(TripTime) -> Mux1/1
  [Iabc_B575_1] -> Protection System1/2(Iabc (pu))
  [wr1] -> Protection System1/5(Speed (pu))
  [Vabc_B575_1] -> Protection System1/1(Vabc (pu))
  Protection System1/3(TripStatus) -> TripData1/1
  Ground2/1 -> Protection System1/4(Reset)
  Ground3/1 -> Protection System2/3(Vdc (V))
  Protection System2/1(Trip) -> Mux/2
  [Iabc_B575_2] -> Protection System2/2(Iabc (pu))
  [wr2] -> Protection System2/5(Speed (pu))
  [Vabc_B575_2] -> Protection System2/1(Vabc (pu))
  Protection System2/3(TripStatus) -> TripData2/1
  Ground4/1 -> Protection System2/4(Reset)
  Ground5/1 -> Protection System3/3(Vdc (V))
  Protection System3/2(TripTime) -> Mux1/3
  Protection System3/1(Trip) -> Mux/3
  [Iabc_B575_3] -> Protection System3/2(Iabc (pu))
  [wr3] -> Protection System3/5(Speed (pu))
  [Vabc_B575_3] -> Protection System3/1(Vabc (pu))
  Protection System3/3(TripStatus) -> TripData3/1
  Ground6/1 -> Protection System3/4(Reset)
  Protection System1/1(Trip) -> Mux/1
  Mux/1 -> Trip1_3/1
  Mux1/1 -> Trip Time1_3/1
  Protection System2/2(TripTime) -> Mux1/2

== system power_wind/Wind Farm 1 & 2 Data acquisition/Mean Value3 ==
  note: Mean value
  In : Inport
  Init : Inport  Port=2
  Gain : Gain  Gain=1/Period  SaturateOnIntegerOverflow=on  OutDataTypeStr=Inherit: Same as input  ParamDataTypeStr=Inherit: Same as input
  Step : Step  Time=Period+eps  SampleTime=0
  Sum : Sum  Inputs=+-  SaturateOnIntegerOverflow=on  InputSameDT=on  OutDataTypeStr=Inherit: Same as first input
  Switch : Switch  Threshold=0.5  SaturateOnIntegerOverflow=on
  Transport Delay : TransportDelay  DelayTime=Period
  integrator : Integrator
  Mean : Outport
  wires:
  Init/1 -> Switch/3
  Step/1 -> Switch/2
  Switch/1 -> Mean/1
  Gain/1 -> Switch/1
  Sum/1 -> Gain/1
  In/1 -> integrator/1
  integrator/1 -> Sum/1, Transport Delay/1
  Transport Delay/1 -> Sum/2

== system power_wind/Wind Farm 1 & 2 Data acquisition/Mean Value4 ==
  note: Mean value
  In : Inport
  Init : Inport  Port=2
  Gain : Gain  Gain=1/Period  SaturateOnIntegerOverflow=on  OutDataTypeStr=Inherit: Same as input  ParamDataTypeStr=Inherit: Same as input
  Step : Step  Time=Period+eps  SampleTime=0
  Sum : Sum  Inputs=+-  SaturateOnIntegerOverflow=on  InputSameDT=on  OutDataTypeStr=Inherit: Same as first input
  Switch : Switch  Threshold=0.5  SaturateOnIntegerOverflow=on
  Transport Delay : TransportDelay  DelayTime=Period
  integrator : Integrator
  Mean : Outport
  wires:
  Transport Delay/1 -> Sum/2
  integrator/1 -> Transport Delay/1, Sum/1
  In/1 -> integrator/1
  Sum/1 -> Gain/1
  Gain/1 -> Switch/1
  Switch/1 -> Mean/1
  Step/1 -> Switch/2
  Init/1 -> Switch/3

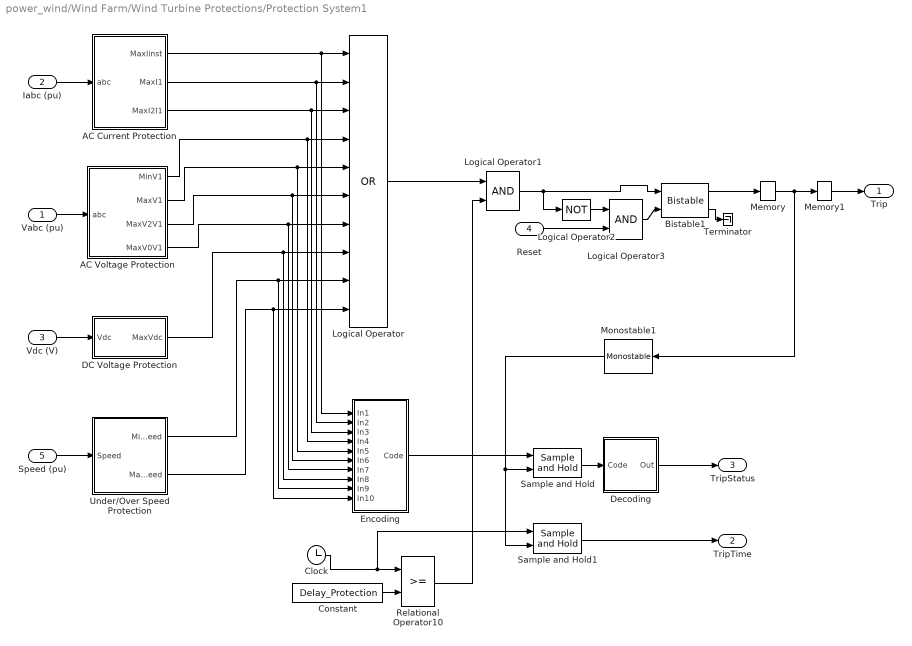
== system power_wind/Wind Farm/Wind Turbine Protections/Protection System1 ==
  Vabc (pu) : Inport  PortDimensions=3
  Iabc (pu) : Inport  Port=2  PortDimensions=3
  Vdc (V) : Inport  Port=3  PortDimensions=1
  Reset : Inport  Port=4  PortDimensions=1
  Speed (pu) : Inport  Port=5  PortDimensions=1
  AC Current Protection : Subsystem
  AC Voltage Protection : Subsystem
  Bistable1 : powerlib_meascontrol/Logic/Bistable  Qpriority=Set  ic=0  Ts=0
  Clock : Clock
  Constant : Constant  Value=Delay_Protection
  DC Voltage Protection : Subsystem
  Decoding : Subsystem
  Encoding : Subsystem
  Logical Operator : Logic  Operator=OR  Inputs=10  AllPortsSameDT=off
  Logical Operator1 : Logic  AllPortsSameDT=off
  Logical Operator2 : Logic  Operator=NOT  AllPortsSameDT=off
  Logical Operator3 : Logic  AllPortsSameDT=off
  Memory : Memory  InheritSampleTime=on
  Memory1 : Memory  InheritSampleTime=on
  Monostable1 : powerlib_meascontrol/Logic/Monostable  EdgeDetect=Rising  PulseDuration=1e-9  ic=0  Ts=0
  Relational Operator10 : RelationalOperator
  Sample and Hold : powerlib_meascontrol/Additional Components/Sample and Hold  ic=0  Ts=0
  Sample and Hold1 : powerlib_meascontrol/Additional Components/Sample and Hold  ic=0  Ts=0
  Terminator : Terminator
  Under/Over Speed Protection : Subsystem
  Trip : Outport
  TripTime : Outport  Port=2
  TripStatus : Outport  Port=3
  wires:
  Memory1/1 -> Trip/1
  Vdc (V)/1 -> DC Voltage Protection/1(Vdc)
  DC Voltage Protection/1(MaxVdc) -> Logical Operator/8, Encoding/8(In8)
  Logical Operator2/1 -> Logical Operator3/1
  Reset/1 -> Logical Operator3/2
  Logical Operator3/1 -> Bistable1/2
  Logical Operator1/1 -> Bistable1/1, Logical Operator2/1
  Encoding/1(Code) -> Sample and Hold/1
  Bistable1/1 -> Memory/1
  Memory/1 -> Monostable1/1, Memory1/1
  Bistable1/2 -> Terminator/1
  Sample and Hold/1 -> Decoding/1(Code)
  Decoding/1(Out) -> TripStatus/1
  Iabc (pu)/1 -> AC Current Protection/1(abc)
  Vabc (pu)/1 -> AC Voltage Protection/1(abc)
  AC Current Protection/1(MaxIinst) -> Logical Operator/1, Encoding/1(In1)
  AC Current Protection/2(MaxI1) -> Logical Operator/2, Encoding/2(In2)
  AC Current Protection/3(MaxI2I1) -> Logical Operator/3, Encoding/3(In3)
  AC Voltage Protection/1(MinV1) -> Logical Operator/4, Encoding/4(In4)
  AC Voltage Protection/2(MaxV1) -> Logical Operator/5, Encoding/5(In5)
  AC Voltage Protection/3(MaxV2V1) -> Logical Operator/6, Encoding/6(In6)
  AC Voltage Protection/4(MaxV0V1) -> Logical Operator/7, Encoding/7(In7)
  Sample and Hold1/1 -> TripTime/1
  Monostable1/1 -> Sample and Hold1/2, Sample and Hold/2
  Constant/1 -> Relational Operator10/2
  Clock/1 -> Sample and Hold1/1, Relational Operator10/1
  Logical Operator/1 -> Logical Operator1/1
  Relational Operator10/1 -> Logical Operator1/2
  Under/Over Speed Protection/1(MinSpeed) -> Logical Operator/9, Encoding/9(In9)
  Under/Over Speed Protection/2(MaxSpeed) -> Logical Operator/10, Encoding/10(In10)
  Speed (pu)/1 -> Under/Over Speed Protection/1(Speed)

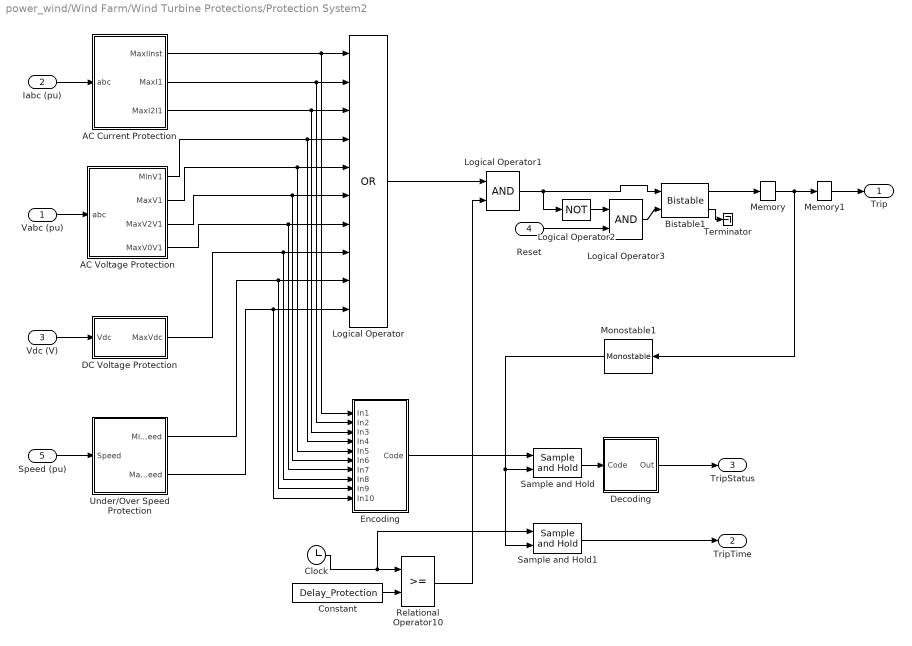
== system power_wind/Wind Farm/Wind Turbine Protections/Protection System2 ==
  Vabc (pu) : Inport  PortDimensions=3
  Iabc (pu) : Inport  Port=2  PortDimensions=3
  Vdc (V) : Inport  Port=3  PortDimensions=1
  Reset : Inport  Port=4  PortDimensions=1
  Speed (pu) : Inport  Port=5  PortDimensions=1
  AC Current Protection : Subsystem
  AC Voltage Protection : Subsystem
  Bistable1 : powerlib_meascontrol/Logic/Bistable  Qpriority=Set  ic=0  Ts=0
  Clock : Clock
  Constant : Constant  Value=Delay_Protection
  DC Voltage Protection : Subsystem
  Decoding : Subsystem
  Encoding : Subsystem
  Logical Operator : Logic  Operator=OR  Inputs=10  AllPortsSameDT=off
  Logical Operator1 : Logic  AllPortsSameDT=off
  Logical Operator2 : Logic  Operator=NOT  AllPortsSameDT=off
  Logical Operator3 : Logic  AllPortsSameDT=off
  Memory : Memory  InheritSampleTime=on
  Memory1 : Memory  InheritSampleTime=on
  Monostable1 : powerlib_meascontrol/Logic/Monostable  EdgeDetect=Rising  PulseDuration=1e-9  ic=0  Ts=0
  Relational Operator10 : RelationalOperator
  Sample and Hold : powerlib_meascontrol/Additional Components/Sample and Hold  ic=0  Ts=0
  Sample and Hold1 : powerlib_meascontrol/Additional Components/Sample and Hold  ic=0  Ts=0
  Terminator : Terminator
  Under/Over Speed Protection : Subsystem
  Trip : Outport
  TripTime : Outport  Port=2
  TripStatus : Outport  Port=3
  wires:
  Speed (pu)/1 -> Under/Over Speed Protection/1(Speed)
  Under/Over Speed Protection/2(MaxSpeed) -> Encoding/10(In10), Logical Operator/10
  Under/Over Speed Protection/1(MinSpeed) -> Encoding/9(In9), Logical Operator/9
  Relational Operator10/1 -> Logical Operator1/2
  Logical Operator/1 -> Logical Operator1/1
  Clock/1 -> Relational Operator10/1, Sample and Hold1/1
  Constant/1 -> Relational Operator10/2
  Monostable1/1 -> Sample and Hold/2, Sample and Hold1/2
  Sample and Hold1/1 -> TripTime/1
  AC Voltage Protection/4(MaxV0V1) -> Encoding/7(In7), Logical Operator/7
  AC Voltage Protection/3(MaxV2V1) -> Encoding/6(In6), Logical Operator/6
  AC Voltage Protection/2(MaxV1) -> Encoding/5(In5), Logical Operator/5
  AC Voltage Protection/1(MinV1) -> Encoding/4(In4), Logical Operator/4
  AC Current Protection/3(MaxI2I1) -> Encoding/3(In3), Logical Operator/3
  AC Current Protection/2(MaxI1) -> Encoding/2(In2), Logical Operator/2
  AC Current Protection/1(MaxIinst) -> Encoding/1(In1), Logical Operator/1
  Vabc (pu)/1 -> AC Voltage Protection/1(abc)
  Iabc (pu)/1 -> AC Current Protection/1(abc)
  Decoding/1(Out) -> TripStatus/1
  Sample and Hold/1 -> Decoding/1(Code)
  Bistable1/2 -> Terminator/1
  Memory/1 -> Memory1/1, Monostable1/1
  Bistable1/1 -> Memory/1
  Encoding/1(Code) -> Sample and Hold/1
  Logical Operator1/1 -> Logical Operator2/1, Bistable1/1
  Logical Operator3/1 -> Bistable1/2
  Reset/1 -> Logical Operator3/2
  Logical Operator2/1 -> Logical Operator3/1
  DC Voltage Protection/1(MaxVdc) -> Encoding/8(In8), Logical Operator/8
  Vdc (V)/1 -> DC Voltage Protection/1(Vdc)
  Memory1/1 -> Trip/1

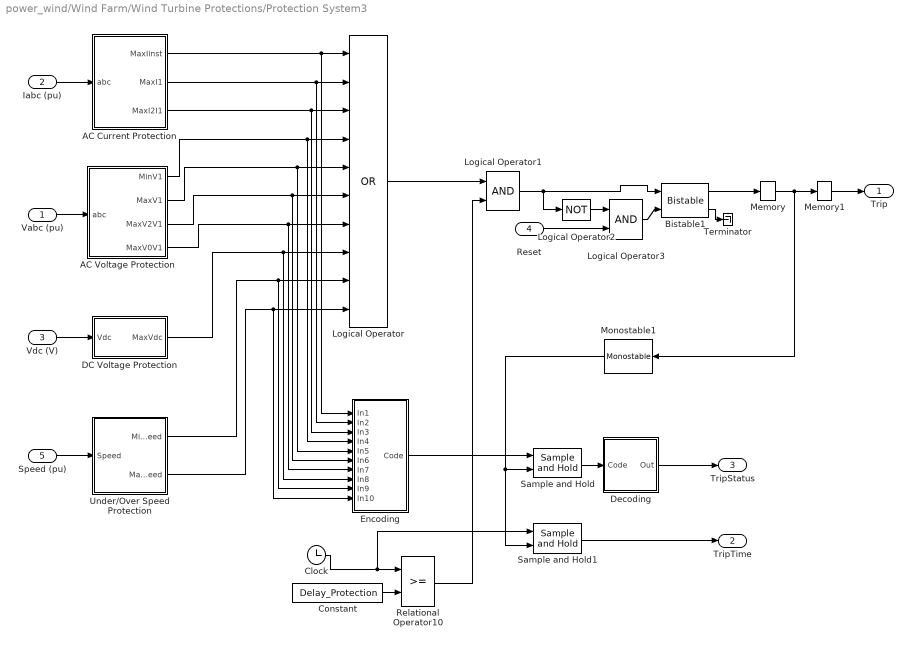
== system power_wind/Wind Farm/Wind Turbine Protections/Protection System3 ==
  Vabc (pu) : Inport  PortDimensions=3
  Iabc (pu) : Inport  Port=2  PortDimensions=3
  Vdc (V) : Inport  Port=3  PortDimensions=1
  Reset : Inport  Port=4  PortDimensions=1
  Speed (pu) : Inport  Port=5  PortDimensions=1
  AC Current Protection : Subsystem
  AC Voltage Protection : Subsystem
  Bistable1 : powerlib_meascontrol/Logic/Bistable  Qpriority=Set  ic=0  Ts=0
  Clock : Clock
  Constant : Constant  Value=Delay_Protection
  DC Voltage Protection : Subsystem
  Decoding : Subsystem
  Encoding : Subsystem
  Logical Operator : Logic  Operator=OR  Inputs=10  AllPortsSameDT=off
  Logical Operator1 : Logic  AllPortsSameDT=off
  Logical Operator2 : Logic  Operator=NOT  AllPortsSameDT=off
  Logical Operator3 : Logic  AllPortsSameDT=off
  Memory : Memory  InheritSampleTime=on
  Memory1 : Memory  InheritSampleTime=on
  Monostable1 : powerlib_meascontrol/Logic/Monostable  EdgeDetect=Rising  PulseDuration=1e-9  ic=0  Ts=0
  Relational Operator10 : RelationalOperator
  Sample and Hold : powerlib_meascontrol/Additional Components/Sample and Hold  ic=0  Ts=0
  Sample and Hold1 : powerlib_meascontrol/Additional Components/Sample and Hold  ic=0  Ts=0
  Terminator : Terminator
  Under/Over Speed Protection : Subsystem
  Trip : Outport
  TripTime : Outport  Port=2
  TripStatus : Outport  Port=3
  wires:
  Memory1/1 -> Trip/1
  Vdc (V)/1 -> DC Voltage Protection/1(Vdc)
  DC Voltage Protection/1(MaxVdc) -> Logical Operator/8, Encoding/8(In8)
  Logical Operator2/1 -> Logical Operator3/1
  Reset/1 -> Logical Operator3/2
  Logical Operator3/1 -> Bistable1/2
  Logical Operator1/1 -> Bistable1/1, Logical Operator2/1
  Encoding/1(Code) -> Sample and Hold/1
  Bistable1/1 -> Memory/1
  Memory/1 -> Monostable1/1, Memory1/1
  Bistable1/2 -> Terminator/1
  Sample and Hold/1 -> Decoding/1(Code)
  Decoding/1(Out) -> TripStatus/1
  Iabc (pu)/1 -> AC Current Protection/1(abc)
  Vabc (pu)/1 -> AC Voltage Protection/1(abc)
  AC Current Protection/1(MaxIinst) -> Logical Operator/1, Encoding/1(In1)
  AC Current Protection/2(MaxI1) -> Logical Operator/2, Encoding/2(In2)
  AC Current Protection/3(MaxI2I1) -> Logical Operator/3, Encoding/3(In3)
  AC Voltage Protection/1(MinV1) -> Logical Operator/4, Encoding/4(In4)
  AC Voltage Protection/2(MaxV1) -> Logical Operator/5, Encoding/5(In5)
  AC Voltage Protection/3(MaxV2V1) -> Logical Operator/6, Encoding/6(In6)
  AC Voltage Protection/4(MaxV0V1) -> Logical Operator/7, Encoding/7(In7)
  Sample and Hold1/1 -> TripTime/1
  Monostable1/1 -> Sample and Hold1/2, Sample and Hold/2
  Constant/1 -> Relational Operator10/2
  Clock/1 -> Sample and Hold1/1, Relational Operator10/1
  Logical Operator/1 -> Logical Operator1/1
  Relational Operator10/1 -> Logical Operator1/2
  Under/Over Speed Protection/1(MinSpeed) -> Logical Operator/9, Encoding/9(In9)
  Under/Over Speed Protection/2(MaxSpeed) -> Logical Operator/10, Encoding/10(In10)
  Speed (pu)/1 -> Under/Over Speed Protection/1(Speed)

== system power_wind/Wind Farm/Wind Turbine Protections/Protection System1/AC Current Protection ==
  abc : Inport  PortDimensions=3
  Complex to Magnitude-Angle1 : ComplexToMagnitudeAngle  Output=Magnitude
  Current Measurement : Subsystem
  MinMax : MinMax  Function=max  ZeroCross=off  SaturateOnIntegerOverflow=on  InputSameDT=on
  Mux : Mux  Inputs=3
  On Delay : powerlib_meascontrol/Logic/On Delay  DelayType=On delay  delay=Delay_I1  ic=0  Ts=0
  On Delay1 : powerlib_meascontrol/Logic/On Delay  DelayType=On delay  delay=Delay_I2_I1  ic=0  Ts=0
  Relational Operator10 : RelationalOperator  Operator=>
  Relational Operator6 : RelationalOperator  Operator=>
  Relational Operator8 : RelationalOperator  Operator=>
  Selector : Selector  InputPortWidth=3
  Selector1 : Selector  InputPortWidth=3  Indices=2
  Selector2 : Selector  InputPortWidth=3  Indices=3
  V0/V1 max3 : Constant  Value=Max_I1
  V1 max : Constant  Value=Max_I2_I1
  V1 max2 : Constant  Value=Max_Iinst
  MaxIinst : Outport
  MaxI1 : Outport  Port=2
  MaxI2I1 : Outport  Port=3
  wires:
  MinMax/1 -> Relational Operator10/1
  Complex to Magnitude-Angle1/1 -> MinMax/1
  Mux/1 -> Complex to Magnitude-Angle1/1
  Selector1/1 -> Mux/2
  Selector2/1 -> Mux/3
  Selector/1 -> Mux/1
  V1 max2/1 -> Relational Operator10/2
  Relational Operator10/1 -> MaxIinst/1
  On Delay1/1 -> MaxI2I1/1
  On Delay/1 -> MaxI1/1
  Relational Operator8/1 -> On Delay1/1
  Relational Operator6/1 -> On Delay/1
  Current Measurement/2(I2/I1) -> Relational Operator8/1
  V1 max/1 -> Relational Operator8/2
  V0/V1 max3/1 -> Relational Operator6/2
  Current Measurement/1(I1) -> Relational Operator6/1
  abc/1 -> Selector2/1, Selector1/1, Selector/1, Current Measurement/1(abc)

== system power_wind/Wind Farm/Wind Turbine Protections/Protection System1/AC Voltage Protection ==
  abc : Inport  PortDimensions=3
  On Delay : powerlib_meascontrol/Logic/On Delay  DelayType=On delay  delay=Delay_V1  ic=0  Ts=0
  On Delay1 : powerlib_meascontrol/Logic/On Delay  DelayType=On delay  delay=Delay_V1  ic=0  Ts=0
  On Delay2 : powerlib_meascontrol/Logic/On Delay  DelayType=On delay  delay=Delay_V2_V1  ic=0  Ts=0
  On Delay3 : powerlib_meascontrol/Logic/On Delay  DelayType=On delay  delay=Delay_V2_V1  ic=0  Ts=0
  Relational Operator6 : RelationalOperator  Operator=>
  Relational Operator7 : RelationalOperator  Operator=<
  Relational Operator8 : RelationalOperator  Operator=>
  Relational Operator9 : RelationalOperator  Operator=>
  V0/V1 max3 : Constant  Value=Max_V1
  V0/V1 max4 : Constant  Value=Min_V1
  V1 max : Constant  Value=Max_V2_V1
  V1 max1 : Constant  Value=Max_V0_V1
  Voltage Measurement : Subsystem
  MinV1 : Outport
  MaxV1 : Outport  Port=2
  MaxV2V1 : Outport  Port=3
  MaxV0V1 : Outport  Port=4
  wires:
  abc/1 -> Voltage Measurement/1(abc)
  Voltage Measurement/1(V1) -> Relational Operator6/1, Relational Operator7/1
  V0/V1 max3/1 -> Relational Operator6/2
  V0/V1 max4/1 -> Relational Operator7/2
  V1 max/1 -> Relational Operator8/2
  Voltage Measurement/2(V2/V1) -> Relational Operator8/1
  V1 max1/1 -> Relational Operator9/2
  Voltage Measurement/3(V0/V1) -> Relational Operator9/1
  Relational Operator6/1 -> On Delay1/1
  Relational Operator7/1 -> On Delay/1
  Relational Operator8/1 -> On Delay2/1
  Relational Operator9/1 -> On Delay3/1
  On Delay1/1 -> MaxV1/1
  On Delay/1 -> MinV1/1
  On Delay2/1 -> MaxV2V1/1
  On Delay3/1 -> MaxV0V1/1

== system power_wind/Wind Farm/Wind Turbine Protections/Protection System1/DC Voltage Protection ==
  Vdc : Inport
  On Delay : powerlib_meascontrol/Logic/On Delay  DelayType=On delay  delay=Delay_Vdc  ic=0  Ts=0
  Relational Operator1 : RelationalOperator  Operator=>
  V1 max3 : Constant  Value=Max_Vdc
  MaxVdc : Outport
  wires:
  On Delay/1 -> MaxVdc/1
  Relational Operator1/1 -> On Delay/1
  V1 max3/1 -> Relational Operator1/2
  Vdc/1 -> Relational Operator1/1
